simulink model "altitude_iLQR"  (R2024a)
settings: Solver=FixedStepAuto  StartTime=0.0  StopTime=SIMTIME  FixedStep=sample_time  RelTol=1e-3
undefined symbols (not defined in the file): A, B, C, K, Ki, u0, y0
settings Model: Creator=Lorenzo-Desk  LastModifiedBy=Lorenzo-Desk

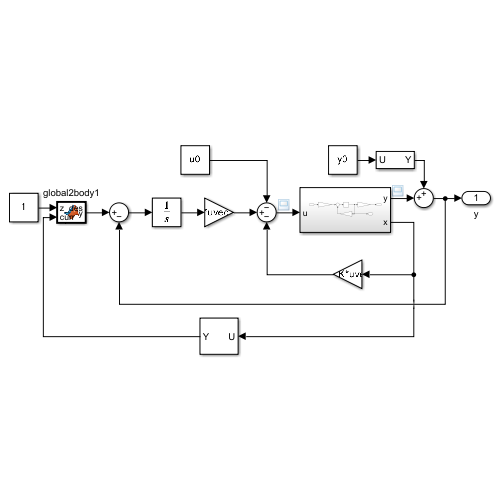
[thumbnail: Simulink's stored preview of the top-level diagram]
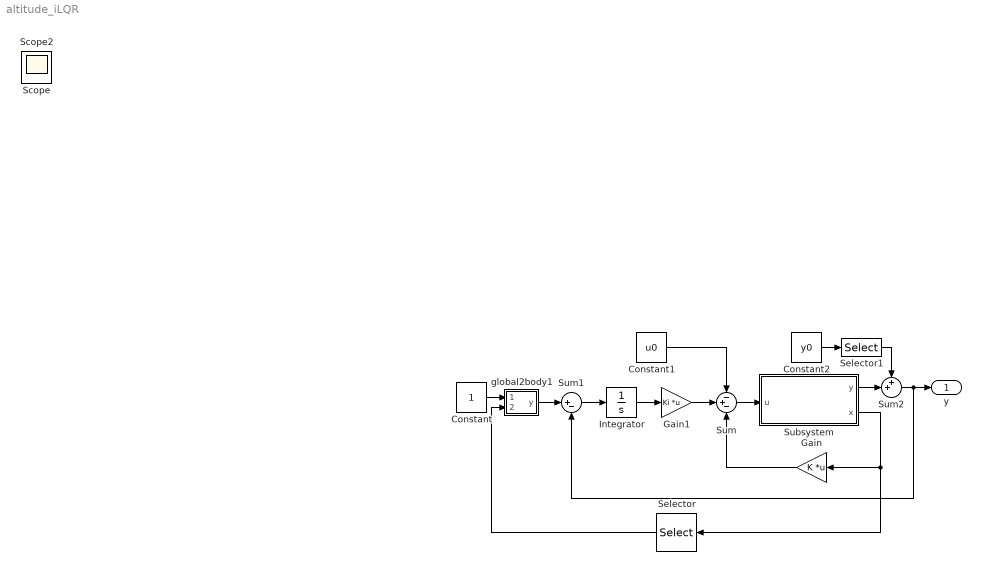
== system altitude_iLQR ==
  Constant : Constant
  Constant1 : Constant  Value=u0
  Constant2 : Constant  Value=y0
  Gain : Gain  Gain=K  Multiplication=Matrix(K*u) (u vector)
  Gain1 : Gain  Gain=Ki  Multiplication=Matrix(K*u) (u vector)
  Integrator : Integrator
  Selector : Selector  InputPortWidth=12  IndexOptions=Index vector (dialog)  Indices=[1 2 3 7 8 9]  OutputSizes=1
  Selector1 : Selector  InputPortWidth=12  IndexOptions=Index vector (dialog)  Indices=[3]  OutputSizes=1
  Subsystem : Subsystem
  Sum : Sum  Inputs=-+-
  Sum1 : Sum  Inputs=|+-
  Sum2 : Sum  Inputs=++|
  global2body1 : MATLAB Function  TreatAsAtomicUnit=on
  y : Outport
  Scope : Scope
  Scope2 : Scope
  wires:
  Sum/1 -> Subsystem/1(u)
  Subsystem/2(x) -> Selector/1, Gain/1
  Sum1/1 -> Integrator/1
  Integrator/1 -> Gain1/1
  Constant/1 -> global2body1/1(z_des)
  global2body1/1(y) -> Sum1/1
  Selector/1 -> global2body1/2(curr)
  Gain/1 -> Sum/3
  Gain1/1 -> Sum/2
  Constant1/1 -> Sum/1
  Sum2/1 -> Sum1/2, y/1
  Subsystem/1(y) -> Sum2/2
  Constant2/1 -> Selector1/1
  Selector1/1 -> Sum2/1

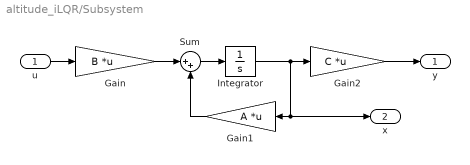
== system altitude_iLQR/Subsystem ==
  u : Inport
  Gain : Gain  Gain=B  Multiplication=Matrix(K*u) (u vector)
  Gain1 : Gain  Gain=A  Multiplication=Matrix(K*u) (u vector)
  Gain2 : Gain  Gain=C  Multiplication=Matrix(K*u) (u vector)
  Integrator : Integrator
  Sum : Sum  Inputs=|++
  y : Outport
  x : Outport  Port=2
  wires:
  u/1 -> Gain/1
  Gain/1 -> Sum/1
  Sum/1 -> Integrator/1
  Gain1/1 -> Sum/2
  Integrator/1 -> Gain2/1, x/1, Gain1/1
  Gain2/1 -> y/1

== matlab function altitude_iLQR/global2body1 ==
  data: z_des input; y output; curr input
function y = fcn(z_des, curr)
pos = curr(1:3); pos(3) = z_des; phi = curr(4); theta = curr(5); psi = curr(6);
% define rotation matrix
R_roll = [...
      1, 0, 0;...
      0, cos(phi), -sin(phi);...
      0, sin(phi), cos(phi)];
R_pitch = [...
      cos(theta), 0, sin(theta);...
      0, 1, 0;...
      -sin(theta), 0, cos(theta)];
R_yaw = [...
      cos(psi), -sin(psi), 0;...
      sin(psi), cos(psi), 0;...
      0, 0, 1];  
  
R = R_yaw*R_pitch*R_roll;

pos = pos'*R;
y = pos(3);
